simulink model "unicycle_kin_trajCont"  (R2020a)
settings: Solver=FixedStepAuto  StartTime=0.0  StopTime=inf  RelTol=1e-3
undefined symbols (not defined in the file or in its folder): Angular, Linear
libraries: robotlib x7

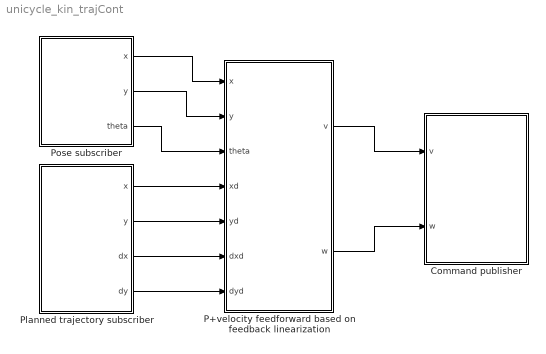
== system unicycle_kin_trajCont ==
  Command publisher : Subsystem  mask{simPublishRate=25}
      mask prompts: simPublishRate "Publising rate [Hz]"
  P+velocity feedforward based on feedback linearization : Subsystem  mask{KP=1.5, epsilon=1}
      mask prompts: KP "Proportional gain"; epsilon "Point P distance"
  Planned trajectory subscriber : Subsystem
  Pose subscriber : Subsystem
  wires:
  P+velocity feedforward based on feedback linearization/1(v) -> Command publisher/1(v)
  P+velocity feedforward based on feedback linearization/2(w) -> Command publisher/2(w)
  Pose subscriber/1(x) -> P+velocity feedforward based on feedback linearization/1(x)
  Pose subscriber/2(y) -> P+velocity feedforward based on feedback linearization/2(y)
  Pose subscriber/3(theta) -> P+velocity feedforward based on feedback linearization/3(theta)
  Planned trajectory subscriber/4(dy) -> P+velocity feedforward based on feedback linearization/7(dyd)
  Planned trajectory subscriber/3(dx) -> P+velocity feedforward based on feedback linearization/6(dxd)
  Planned trajectory subscriber/1(x) -> P+velocity feedforward based on feedback linearization/4(xd)
  Planned trajectory subscriber/2(y) -> P+velocity feedforward based on feedback linearization/5(yd)

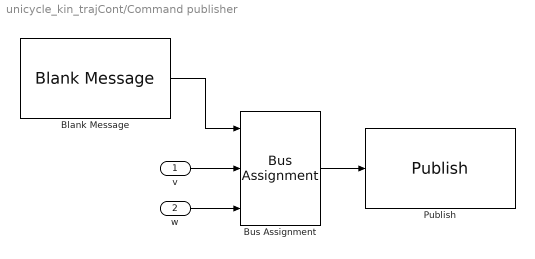
== system unicycle_kin_trajCont/Command publisher ==
  v : Inport  SampleTime=1/simPublishRate
  w : Inport  Port=2  SampleTime=1/simPublishRate
  Blank Message : robotlib/Blank Message  messageClass=Message  entityType=geometry_msgs/Twist  messageType=geometry_msgs/Twist  SampleTime=1/simPublishRate
  Bus Assignment : BusAssignment  AssignedSignals=Linear.X,Angular.Z
  Publish : robotlib/Publish  topicSource=Specify your own  topic=/cmd_vel  messageType=geometry_msgs/Twist  messageQueueLength=1
  wires:
  Bus Assignment/1 -> Publish/1
  Blank Message/1 -> Bus Assignment/1
  v/1 -> Bus Assignment/2
  w/1 -> Bus Assignment/3

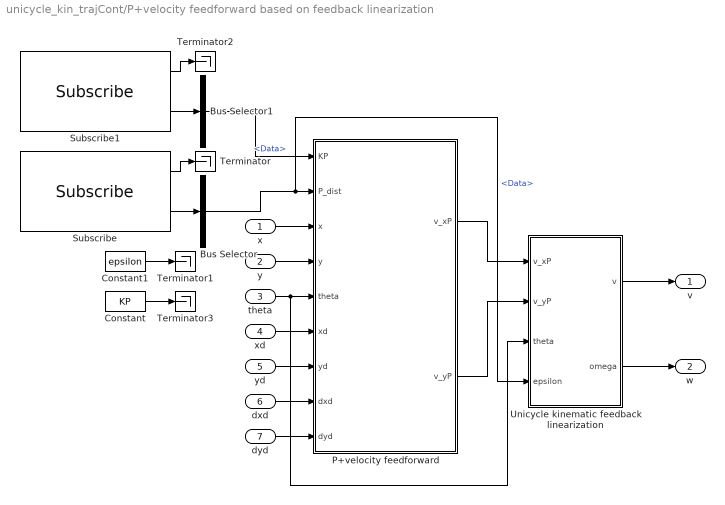
== system unicycle_kin_trajCont/P+velocity feedforward based on feedback linearization ==
  x : Inport
  y : Inport  Port=2
  theta : Inport  Port=3
  xd : Inport  Port=4
  yd : Inport  Port=5
  dxd : Inport  Port=6
  dyd : Inport  Port=7
  Bus Selector : BusSelector  OutputSignals=Data
  Bus Selector1 : BusSelector  OutputSignals=Data
  Constant : Constant  Value=KP
  Constant1 : Constant  Value=epsilon
  P+velocity feedforward : MATLAB Function  TreatAsAtomicUnit=on
  Subscribe : robotlib/Subscribe  topicSource=Specify your own  topic=/epsilon  messageType=std_msgs/Float64  sampleTime=-1  messageQueueLength=1
  Subscribe1 : robotlib/Subscribe  topicSource=Specify your own  topic=/Kp  messageType=std_msgs/Float64  sampleTime=-1  messageQueueLength=1
  Terminator{,1..3} (4 alike) : Terminator
  Unicycle kinematic feedback linearization : Subsystem  mask{epsilon=10}
  v : Outport  VectorParamsAs1DForOutWhenUnconnected=off
  w : Outport  Port=2  VectorParamsAs1DForOutWhenUnconnected=off
  wires:
  dyd/1 -> P+velocity feedforward/9(dyd)
  Bus Selector1/1 -> P+velocity feedforward/1(KP)  "<Data>"
  x/1 -> P+velocity feedforward/3(x)
  y/1 -> P+velocity feedforward/4(y)
  xd/1 -> P+velocity feedforward/6(xd)
  yd/1 -> P+velocity feedforward/7(yd)
  dxd/1 -> P+velocity feedforward/8(dxd)
  P+velocity feedforward/2(v_yP) -> Unicycle kinematic feedback linearization/2(v_yP)
  P+velocity feedforward/1(v_xP) -> Unicycle kinematic feedback linearization/1(v_xP)
  Unicycle kinematic feedback linearization/2(omega) -> w/1
  Unicycle kinematic feedback linearization/1(v) -> v/1
  theta/1 -> Unicycle kinematic feedback linearization/3(theta), P+velocity feedforward/5(theta)
  Subscribe/1 -> Terminator/1
  Constant1/1 -> Terminator1/1
  Subscribe/2 -> Bus Selector/1
  Bus Selector/1 -> Unicycle kinematic feedback linearization/4(epsilon), P+velocity feedforward/2(P_dist)  "<Data>"
  Subscribe1/1 -> Terminator2/1
  Subscribe1/2 -> Bus Selector1/1
  Constant/1 -> Terminator3/1

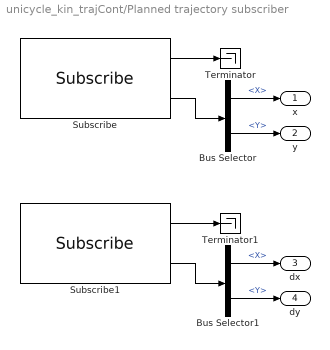
== system unicycle_kin_trajCont/Planned trajectory subscriber ==
  Bus Selector : BusSelector  OutputSignals=X,Y
  Bus Selector1 : BusSelector  OutputSignals=X,Y
  Subscribe : robotlib/Subscribe  topicSource=Specify your own  topic=/desired_position  messageType=geometry_msgs/Point  sampleTime=-1  messageQueueLength=1
  Subscribe1 : robotlib/Subscribe  topicSource=Specify your own  topic=/desired_velocity  messageType=geometry_msgs/Point  sampleTime=-1  messageQueueLength=1
  Terminator : Terminator
  Terminator1 : Terminator
  x : Outport
  y : Outport  Port=2
  dx : Outport  Port=3
  dy : Outport  Port=4
  wires:
  Bus Selector/2 -> y/1  "<Y>"
  Subscribe/1 -> Terminator/1
  Subscribe/2 -> Bus Selector/1
  Bus Selector/1 -> x/1  "<X>"
  Bus Selector1/2 -> dy/1  "<Y>"
  Bus Selector1/1 -> dx/1  "<X>"
  Subscribe1/1 -> Terminator1/1
  Subscribe1/2 -> Bus Selector1/1

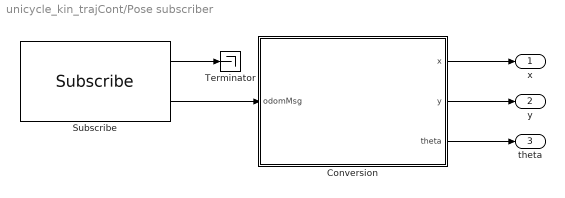
== system unicycle_kin_trajCont/Pose subscriber ==
  Conversion : MATLAB Function  TreatAsAtomicUnit=on
  Subscribe : robotlib/Subscribe  topicSource=Specify your own  topic=/odom  messageType=nav_msgs/Odometry  sampleTime=-1  messageQueueLength=1
  Terminator : Terminator
  x : Outport
  y : Outport  Port=2
  theta : Outport  Port=3
  wires:
  Subscribe/1 -> Terminator/1
  Subscribe/2 -> Conversion/1(odomMsg)
  Conversion/1(x) -> x/1
  Conversion/2(y) -> y/1
  Conversion/3(theta) -> theta/1

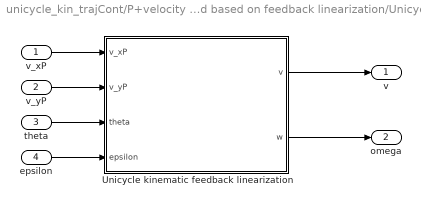
== system unicycle_kin_trajCont/P+velocity feedforward based on feedback linearization/Unicycle kinematic feedback linearization ==
  v_xP : Inport
  v_yP : Inport  Port=2
  theta : Inport  Port=3
  epsilon : Inport  Port=4
  Unicycle kinematic feedback linearization : MATLAB Function  TreatAsAtomicUnit=on
  v : Outport  VectorParamsAs1DForOutWhenUnconnected=off
  omega : Outport  Port=2  VectorParamsAs1DForOutWhenUnconnected=off
  wires:
  Unicycle kinematic feedback linearization/2(w) -> omega/1
  v_yP/1 -> Unicycle kinematic feedback linearization/2(v_yP)
  Unicycle kinematic feedback linearization/1(v) -> v/1
  v_xP/1 -> Unicycle kinematic feedback linearization/1(v_xP)
  theta/1 -> Unicycle kinematic feedback linearization/3(theta)
  epsilon/1 -> Unicycle kinematic feedback linearization/4(epsilon)

== matlab function unicycle_kin_trajCont/P+velocity feedforward based on feedback linearization/Unicycle kinematic feedback linearization/Unicycle kinematic feedback linearization ==
function [v,w] = fblin_unicycle_kinematic(v_xP,v_yP,theta,epsilon)

if(epsilon == 0)
    epsilon = 0.1;
end

v = v_xP*cos(theta)+v_yP*sin(theta);
w = (v_yP*cos(theta)-v_xP*sin(theta))/epsilon;

== matlab function unicycle_kin_trajCont/P+velocity feedforward based on feedback linearization/P+velocity feedforward ==
function [v_xP,v_yP] = P_velFeedforward(KP,P_dist,x,y,theta,xd,yd,dxd,dyd)

if(P_dist == 0)
    P_dist = 0.1;
    KP = 1.5;
end
% Point P transformation
xP = x+P_dist*cos(theta);
yP = y+P_dist*sin(theta);

xPd = xd+P_dist*cos(theta);
yPd = yd+P_dist*sin(theta);

% Control law
v_xP = dxd + KP*(xPd-xP);
v_yP = dyd + KP*(yPd-yP);

== matlab function unicycle_kin_trajCont/Pose subscriber/Conversion ==
function [x,y,theta]  = odom_2_xytheta(odomMsg)

% Position
x = odomMsg.Pose.Pose.Position.X;
y = odomMsg.Pose.Pose.Position.Y;

% Orientation
orientation = [odomMsg.Pose.Pose.Orientation.X,odomMsg.Pose.Pose.Orientation.Y,...
    odomMsg.Pose.Pose.Orientation.Z,odomMsg.Pose.Pose.Orientation.W];

if all(orientation==zeros(1,4))
    theta = 0;
else
    eul = quat2eul(orientation,'ZYX');
    theta = eul(3);
end
